simulink model "vehiclemodel"  (R2020a)
settings: Solver=VariableStepAuto  StartTime=0  StopTime=2400  RelTol=1e-3
values from neighbouring files (symbols this model uses):
  Ctr = 1.6    [ACC_DATA.m]
  F_aero = 1/(2*m_Follower)*Ro_A_Cd    (= 0.00026)    [ACC_DATA.m]
  F_grav = g*sin(theta)    [ACC_DATA.m]
  F_res = g*Cr*cos(theta)    [ACC_DATA.m]
  g = 9.81    [ACC_DATA.m]
  Kb = 0.08    [ACC_DATA.m]
  Kc = 1    [ACC_DATA.m]
  m_Follower = 1500    [ACC_DATA.m]
  r = 0.326    [ACC_DATA.m]
  Rf = 3.28    [ACC_DATA.m]
  Rtr = 1    [ACC_DATA.m]
  Tmax = 528.7 + 0.152*Ne - 0.0000217*Ne^2    (= 789.5)    [ACC_DATA.m]
  Ts = 0.1    [ACC_DATA.m]
  x0_ego = 10    [ACC_DATA.m]
undefined symbols (not defined in the file or in its folder): sigbuilder_block
libraries: autolibshared x2, simulink x1
settings Model: Creator=91968  LastModifiedBy=91968

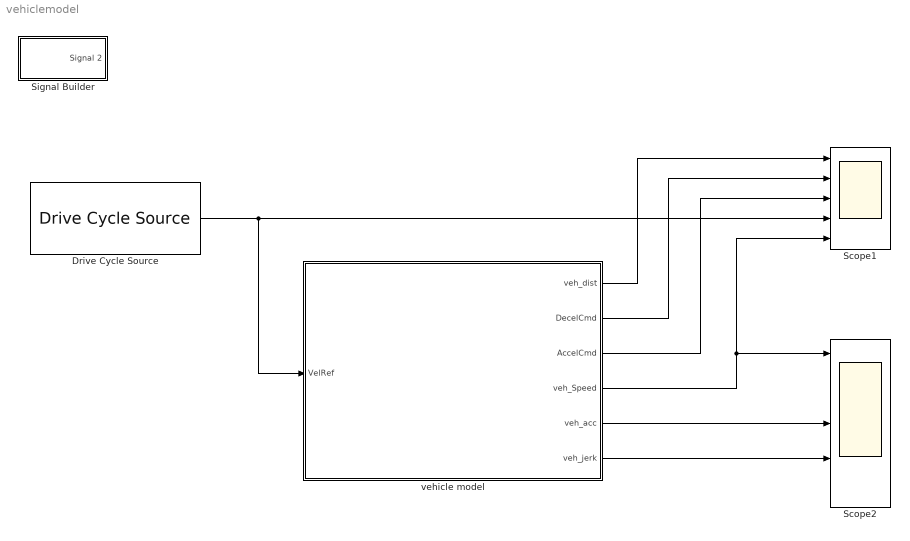
== system vehiclemodel ==
  Drive Cycle Source : autolibshared/Drive Cycle Source  cycleVar=FTP75  fileVar=cycleFTP75.mat  tfinal="2474  seconds"  cycleRepeat=off  outAccPort=off  outGearPort=off  gearList=No gear data  t_wot1=5  xdot_woto=0  xdot_wot1=30  t_wot2=20  xdot_wot2=0  t_wotend=30  srcUnit=m/s  outUnit=m/s  srcAccUnit=m/s/s  outAccUnit=m/s^2  dt=0  aMode=1  faultOption=off  velBnd=2  velBndUnit=mph  inUnit=m/s  timeBnd=1  failOption=off  stopSim=off  maxFaultCnt=10  maxFaultTime=2  maxTotFaultTime=15  traceOption=off  dtTrace=1  traceWindow=10  lastDCname=FTP75 Velocity  lastOutUnit=mph  lastDT=0  lastTB=1  lastSB=2  forceCalcBound=off
      settings: SourceProductBaseCode=PW,MT,VE,VP
  Scope1 : Scope  NumInputPorts=5
  Scope2 : Scope  NumInputPorts=5
  Signal Builder : Subsystem  Tag=STV Subsys  LoadFcn=sigbuilder_block('load');  StartFcn=sigbuilder_block('start');  StopFcn=sigbuilder_block('stop');  ClipboardFcn=sigbuilder_block('clipboard');  mask(Sigbuilder block){tuvar=[0:10]}
      mask help: Simulink:masks:SigbuilderBlock_MD
      mask init:
      | if ~strcmp(get_param(bdroot(gcbh),'SimulationStatus'),'stopped') tuvar = sigbuilder_block('maskInit'); end
      settings: CopyFcn=sigbuilder_block('copy');  DeleteFcn=sigbuilder_block('delete');  ModelCloseFcn=sigbuilder_block('modelClose');  PreSaveFcn=sigbuilder_block('preSave');  PauseFcn=sigbuilder_block('pause');  ContinueFcn=sigbuilder_block('continue');  NameChangeFcn=sigbuilder_block('namechange');  OpenFcn=sigbuilder_block('open',[437.6 199.2 550.4 400 ]);  CloseFcn=sigbuilder_block('close');
      mask Display: plot(0, 0, 100, 100,[2, 2, 32, 32, 2], [68, 8, 8, 68, 68],[32, 2], [38, 38], [32, 19, 2],[53, 60, 44], [32, 17, 17, 2],[16, 16, 31, 31]);txt = getActiveGroup(gcbh);text(2, 100, txt,'verticalAlignment', 'top');
  vehicle model : Subsystem
      mask Display: image('Volvo-S60-130220211541.jpg'); % Use "Edit Image" on toolstrip to change.
  wires:
  Drive Cycle Source/1 -> Scope1/4, vehicle model/1(VelRef)
  vehicle model/4(veh_Speed) -> Scope1/5, Scope2/1
  vehicle model/1(veh_dist) -> Scope1/1
  vehicle model/2(DecelCmd) -> Scope1/2
  vehicle model/3(AccelCmd) -> Scope1/3
  vehicle model/5(veh_acc) -> Scope2/3
  vehicle model/6(veh_jerk) -> Scope2/4

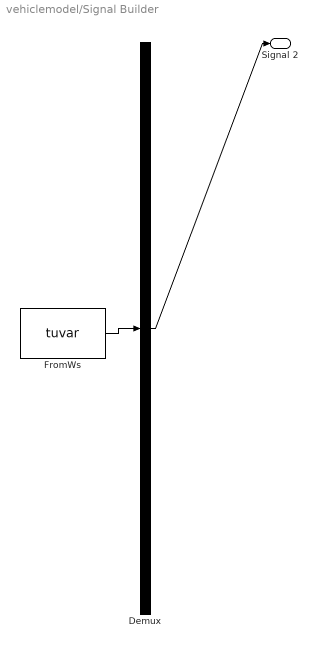
== system vehiclemodel/Signal Builder ==
  Demux : Demux  Tag=STV Demux  Outputs=1
      settings: DisplayOption=none
  FromWs : FromWorkspace  Tag=STV FromWs  VariableName=tuvar
      SigBuilderData=|
      | common.afterFinalStr = 'Extrapolate'
      | common.sampleTime = 0
      | dataSet.timeRange = [0 1000]
      | dataSet.name = 'Group 1'
      | sbobj.Groups.Name = 'Group 1'
      | sbobj.Groups.Signals.Name = 'Signal 2'
      | sbobj.Groups.Signals.XData = [0 3 4 6 6.48 7 7.98 10 102 204 298 400 506 602 700 800 898 1000]
      | sbobj.Groups.Signals.YData = [0 0 0 0 0 10 10 20 20 30 35 20 15 15 12 10 35 20]
      | sbobj.Groups.TimeRange = [0 1000]
  Signal 2 : Outport  Tag=STV Outport
  wires:
  FromWs/1 -> Demux/1
  Demux/1 -> Signal 2/1

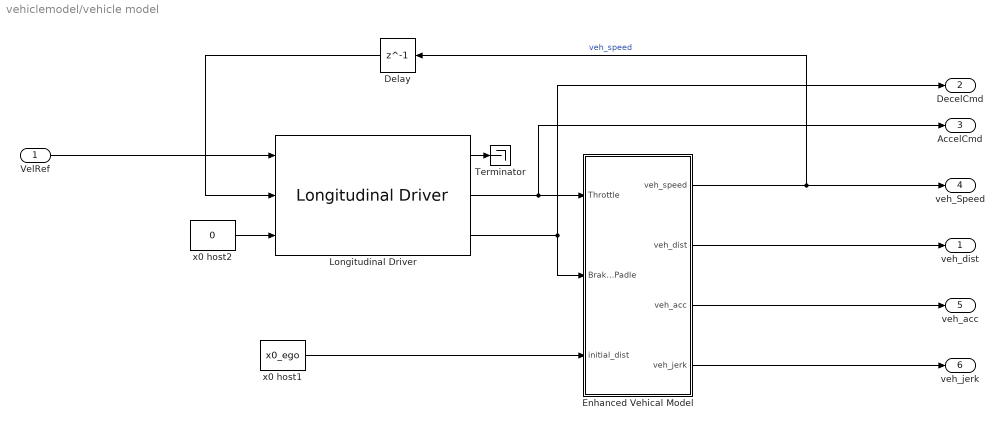
== system vehiclemodel/vehicle model ==
  VelRef : Inport
  Delay : Delay  DelayLength=1  InitialCondition=0
  Enhanced Vehical Model : Subsystem
  Longitudinal Driver : autolibshared/Longitudinal Driver  extAccelOvr=off  extDecelOvr=off  extAccelHld=off  extDecelHld=off  extAccelZero=off  extDecelZero=off  cntrlType=PI  shftType=None  velUnits=m/s  gearOut=off  Kp=15  Ki=1  Kff=.05  Kg=.01  VehVelVec=[0 100]  KffVec=[.1 .1]  KpVec=[10 10]  KiVec=[5 5]  KgVec=[0 0]  m=1500  Kpt=3000  tau=.1  L=2  aR=200  bR=2.5  cR=.5  g=9.81  vnom=100  Kaw=.1  tauerr=.03  tauPt=2  GearInit=0  tShift=.1  pdlVec=[0.1 0.4 0.5 0.9]  upShftTbl=[-1 12.9375 26.4375 39.9375 51.18749999999999 62.4375 72.84375 83.25;-1 16.3125 29.8125 43.3125 54.5624 65.8125 76.78125 87.75;-1 19.6875 33.1875 46.68749999999999 57.9375 69.1875 80.71875 92.25;-1 33 52.5 77.25 100.5 138.75 161.875 185]  dwnShftTbl=[1 9.5625 23.0625 36.5625 47.8125 59.0625 68.90625 78.75;1 12.9375 26.4375 39.9375 51.18749999999999 62.4375 72.84375 83.25;1 16.3125 29.8125 43.3125 54.562499 65.8125 76.78125 87.75;1 19.6875 33.1875 46.68749999999999 57.9375 69.1875 80.71875 92.25]  tClutch=.5  tRev=.5  tPark=120  aMode=1  UpGearVec="[0  1  2  3  4  5  6  7]"  DownGearVec="[1  2  3  4  5  6  7  8]"
      settings: SourceProductBaseCode=PW,MT,VE,VP
  Terminator : Terminator
  x0 host1 : Constant  Value=x0_ego  SampleTime=Ts
  x0 host2 : Constant  Value=0  SampleTime=Ts
  veh_dist : Outport
  DecelCmd : Outport  Port=2
  AccelCmd : Outport  Port=3
  veh_Speed : Outport  Port=4
  veh_acc : Outport  Port=5
  veh_jerk : Outport  Port=6
  wires:
  Longitudinal Driver/2 -> AccelCmd/1, Enhanced Vehical Model/1(Throttle)
  VelRef/1 -> Longitudinal Driver/1
  Enhanced Vehical Model/2(veh_dist) -> veh_dist/1
  x0 host1/1 -> Enhanced Vehical Model/3(initial_dist)
  Longitudinal Driver/3 -> DecelCmd/1, Enhanced Vehical Model/2(Brake_Padle)
  Delay/1 -> Longitudinal Driver/2
  x0 host2/1 -> Longitudinal Driver/3
  Enhanced Vehical Model/1(veh_speed) -> Delay/1, veh_Speed/1  "veh_speed"
  Enhanced Vehical Model/4(veh_jerk) -> veh_jerk/1
  Enhanced Vehical Model/3(veh_acc) -> veh_acc/1
  Longitudinal Driver/1 -> Terminator/1

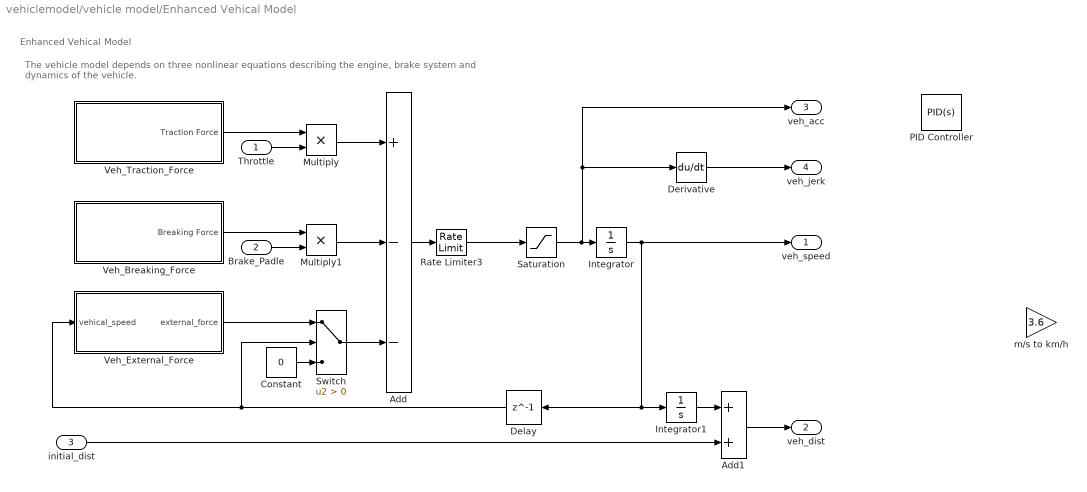
== system vehiclemodel/vehicle model/Enhanced Vehical Model ==
  note: The vehicle model depends on three nonlinear equations describing the engine, brake system and dynamics of the vehicle.
  note: Enhanced Vehical Model
  Throttle : Inport
  Brake_Padle : Inport  Port=2
  initial_dist : Inport  Port=3
  Add : Sum  Inputs=+--
  Add1 : Sum
  Constant : Constant  Value=0
  Delay : Delay  DelayLength=1  InitialCondition=0
  Derivative : Derivative
  Integrator : Integrator
  Integrator1 : Integrator
  Multiply : Product
  Multiply1 : Product
  PID Controller : simulink/Continuous/PID Controller  Controller=PID  Form=Parallel  TimeDomain=Continuous-time  UseExternalTs=off  SampleTime=-1  IntegratorMethod=Forward Euler  FilterMethod=Forward Euler  ControllerParametersSource=internal  P=1  I=1  D=0  UseFilter=on  N=100  TunerSelectOption=Transfer Function Based (PID Tuner App)  InitialConditionSource=internal  InitialConditionForIntegrator=0  InitialConditionForFilter=0  DifferentiatorICPrevScaledInput=0  ExternalReset=none  TrackingMode=off  Kt=1  LimitOutput=off  UpperSaturationLimit=inf  LowerSaturationLimit=-inf  LinearizeAsGain=on  AntiWindupMode=none  Kb=1  POutMin=[]  POutMax=[]  IOutMin=[]  IOutMax=[]  DOutMin=[]  DOutMax=[]  NOutMin=[]  NOutMax=[]  SumOutMin=[]  SumOutMax=[]  SaturationOutMin=[]  SaturationOutMax=[]  PParamMin=[]  PParamMax=[]  IParamMin=[]  IParamMax=[]  DParamMin=[]  DParamMax=[]  NParamMin=[]  NParamMax=[]  KbParamMin=[]  KbParamMax=[]  KtParamMin=[]  KtParamMax=[]  KbOutMin=[]  KbOutMax=[]  KtOutMin=[]  KtOutMax=[]  IntegratorOutMin=[]  IntegratorOutMax=[]  FilterOutMin=[]  FilterOutMax=[]  SumI1OutMin=[]  SumI1OutMax=[]  SumI2OutMin=[]  SumI2OutMax=[]  SumI3OutMin=[]  SumI3OutMax=[]  SumI4OutMin=[]  SumI4OutMax=[]  SumDOutMin=[]  SumDOutMax=[]  DifferentiatorOutMin=[]  DifferentiatorOutMax=[]  FilterDiffOutCoefMin=[]  FilterDiffOutCoefMax=[]  ReciprocalOutMin=[]  ReciprocalOutMax=[]  SumDenOutMin=[]  SumDenOutMax=[]  SumNumOutMin=[]  SumNumOutMax=[]  DivideOutMin=[]  DivideOutMax=[]  UdiffTsProdOutMin=[]  UdiffTsProdOutMax=[]  NTsProdOutMin=[]  NTsProdOutMax=[]  UintegralTsProdOutMin=[]  UintegralTsProdOutMax=[]  UngainTsProdOutMin=[]  UngainTsProdOutMax=[]  IntegratorContinuousStateAttributes=''  IntegratorStateMustResolveToSignalObject=off  IntegratorRTWStateStorageClass=Auto  FilterContinuousStateAttributes=''  FilterStateMustResolveToSignalObject=off  FilterRTWStateStorageClass=Auto  ParallelPVariant=InternalParameters  IdealPVariant=Disabled  IVariant=InternalParameters  DVariant=InternalParameters  IntegratorVariant=Continuous  SatVariant=Disabled  AWVariant=Passthrough  PCopyVariant=Disabled  TRVariant=Disabled  FdbkBlocksVariant=Forward  IdealPFdbkVariant=Disabled  SatFdbkVariant=Disabled  DerivativeFilterVariant=ContFilter  NVariant=InternalParameters  NCopyVariant=Disabled  FilterICVariant=InternalICsFilter  IntegratorICVariant=InternalICs  ExternalResetVariant=Disabled  TRSumVariant=Passthrough  SumFdbkVariant=Disabled  SumVariant=Sum_PID  TsampFilterVariant=InternalTs  TsampNgainVariant=Passthrough  TsampIntegralVariant=Passthrough
  Rate Limiter3 : RateLimiter
  Saturation : Saturate  UpperLimit=3  LowerLimit=-3
  Switch : Switch  Criteria=u2 > Threshold  SaturateOnIntegerOverflow=on  InputSameDT=on
  Veh_Breaking_Force : Subsystem
  Veh_External_Force : Subsystem
  Veh_Traction_Force : Subsystem
  m/s to km/h : Gain  Gain=3.6
  veh_speed : Outport  VectorParamsAs1DForOutWhenUnconnected=off
  veh_dist : Outport  Port=2  VectorParamsAs1DForOutWhenUnconnected=off
  veh_acc : Outport  Port=3  VectorParamsAs1DForOutWhenUnconnected=off
  veh_jerk : Outport  Port=4  VectorParamsAs1DForOutWhenUnconnected=off
  wires:
  Switch/1 -> Add/3
  Brake_Padle/1 -> Multiply1/2
  Veh_Breaking_Force/1("Breaking Force ") -> Multiply1/1
  Throttle/1 -> Multiply/2
  Multiply1/1 -> Add/2
  Multiply/1 -> Add/1
  Veh_Traction_Force/1(Traction Force) -> Multiply/1
  Integrator1/1 -> Add1/1
  Add1/1 -> veh_dist/1
  initial_dist/1 -> Add1/2
  Delay/1 -> Switch/2, Veh_External_Force/1(vehical_speed)
  Veh_External_Force/1(external_force) -> Switch/1
  Constant/1 -> Switch/3
  Add/1 -> Rate Limiter3/1
  Derivative/1 -> veh_jerk/1
  Rate Limiter3/1 -> Saturation/1
  Saturation/1 -> Integrator/1, veh_acc/1, Derivative/1
  Integrator/1 -> veh_speed/1, Delay/1, Integrator1/1

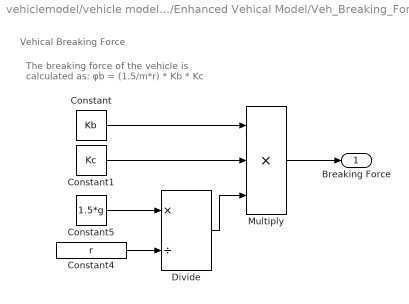
== system vehiclemodel/vehicle model/Enhanced Vehical Model/Veh_Breaking_Force ==
  note: Vehical Breaking Force
  note: The breaking force of the vehicle is calculated as:
      | φb = (1.5/m*r) * Kb * Kc
  Constant : Constant  Value=Kb
  Constant1 : Constant  Value=Kc
  Constant4 : Constant  Value=r
  Constant5 : Constant  Value=1.5*g
  Divide : Product  Inputs=*/
  Multiply : Product  Inputs=3
  "Breaking Force " : Outport  VectorParamsAs1DForOutWhenUnconnected=off
  wires:
  Multiply/1 -> "Breaking Force "/1
  Constant4/1 -> Divide/2
  Constant1/1 -> Multiply/2
  Constant/1 -> Multiply/1
  Constant5/1 -> Divide/1
  Divide/1 -> Multiply/3

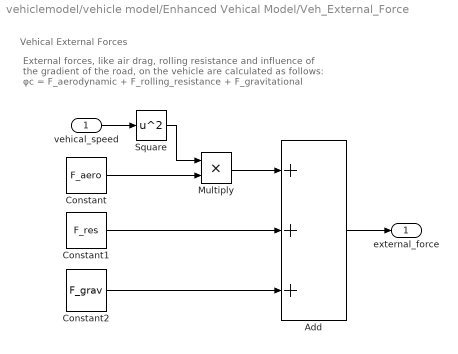
== system vehiclemodel/vehicle model/Enhanced Vehical Model/Veh_External_Force ==
  note: External forces, like air drag, rolling resistance and
      | influence of the gradient of the road, on the vehicle are calculated as follows:
      |
      | φc = F_aerodynamic + F_rolling_resistance + F_gravitational
  note: Vehical External Forces
  vehical_speed : Inport
  Add : Sum  Inputs=+++
  Constant : Constant  Value=F_aero
  Constant1 : Constant  Value=F_res
  Constant2 : Constant  Value=F_grav
  Multiply : Product
  Square : Math  Operator=square  SignedPower=on  SaturateOnIntegerOverflow=on
  external_force : Outport  VectorParamsAs1DForOutWhenUnconnected=off
  wires:
  Add/1 -> external_force/1
  Constant1/1 -> Add/2
  Constant2/1 -> Add/3
  Constant/1 -> Multiply/2
  vehical_speed/1 -> Square/1
  Square/1 -> Multiply/1
  Multiply/1 -> Add/1

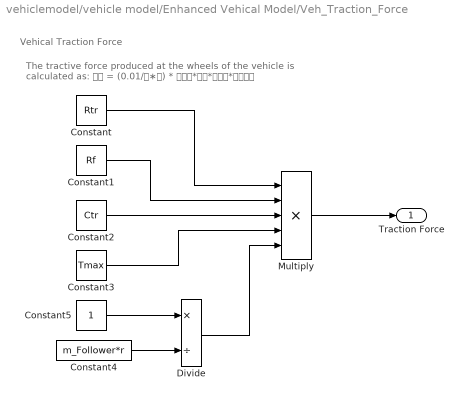
== system vehiclemodel/vehicle model/Enhanced Vehical Model/Veh_Traction_Force ==
  note: The tractive force produced at the wheels of the vehicle is calculated as:
      | 𝜑𝑡 = (0.01/𝑚∗𝑟) * 𝑅𝑡𝑟*𝑅𝑓*𝐶𝑡𝑟*𝑇𝑚𝑎𝑥
  note: Vehical Traction Force
  Constant : Constant  Value=Rtr
  Constant1 : Constant  Value=Rf
  Constant2 : Constant  Value=Ctr
  Constant3 : Constant  Value=Tmax
  Constant4 : Constant  Value=m_Follower*r
  Constant5 : Constant
  Divide : Product  Inputs=*/
  Multiply : Product  Inputs=5
  Traction Force : Outport  VectorParamsAs1DForOutWhenUnconnected=off
  wires:
  Constant/1 -> Multiply/1
  Constant4/1 -> Divide/2
  Constant1/1 -> Multiply/2
  Constant5/1 -> Divide/1
  Constant3/1 -> Multiply/4
  Divide/1 -> Multiply/5
  Constant2/1 -> Multiply/3
  Multiply/1 -> Traction Force/1
